simulink model "TLC_Network"  (R2022b)
settings: Solver=VariableStepAuto  StartTime=0.0  StopTime=2  RelTol=1e-3
(part 2 of 2)

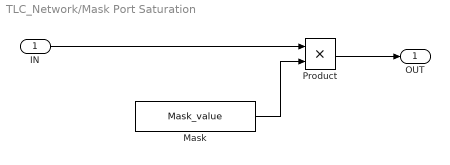
== system TLC_Network/Mask Port Saturation ==
  IN : Inport
  Mask : Constant  Value=Mask_value
  Product : Product
  OUT : Outport
  wires:
  Product/1 -> OUT/1
  IN/1 -> Product/1
  Mask/1 -> Product/2

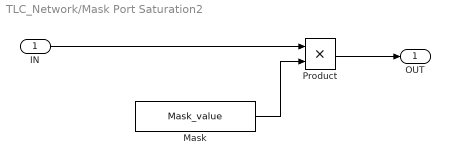
== system TLC_Network/Mask Port Saturation2 ==
  IN : Inport
  Mask : Constant  Value=Mask_value
  Product : Product
  OUT : Outport
  wires:
  Product/1 -> OUT/1
  IN/1 -> Product/1
  Mask/1 -> Product/2

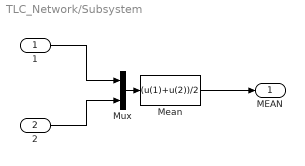
== system TLC_Network/Subsystem ==
  1 : Inport
  2 : Inport  Port=2
  Mean : Fcn  Expr=(u(1)+u(2))/2
  Mux : Mux  Inputs=2
  MEAN : Outport  VectorParamsAs1DForOutWhenUnconnected=off
  wires:
  1/1 -> Mux/1
  Mux/1 -> Mean/1
  2/1 -> Mux/2
  Mean/1 -> MEAN/1

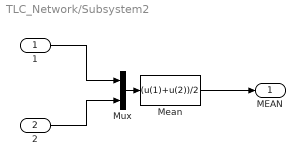
== system TLC_Network/Subsystem2 ==
  1 : Inport
  2 : Inport  Port=2
  Mean : Fcn  Expr=(u(1)+u(2))/2
  Mux : Mux  Inputs=2
  MEAN : Outport  VectorParamsAs1DForOutWhenUnconnected=off
  wires:
  1/1 -> Mux/1
  Mux/1 -> Mean/1
  2/1 -> Mux/2
  Mean/1 -> MEAN/1

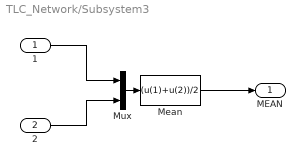
== system TLC_Network/Subsystem3 ==
  1 : Inport
  2 : Inport  Port=2
  Mean : Fcn  Expr=(u(1)+u(2))/2
  Mux : Mux  Inputs=2
  MEAN : Outport  VectorParamsAs1DForOutWhenUnconnected=off
  wires:
  1/1 -> Mux/1
  Mux/1 -> Mean/1
  2/1 -> Mux/2
  Mean/1 -> MEAN/1

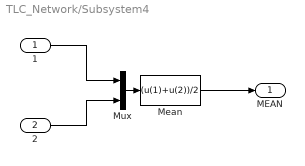
== system TLC_Network/Subsystem4 ==
  1 : Inport
  2 : Inport  Port=2
  Mean : Fcn  Expr=(u(1)+u(2))/2
  Mux : Mux  Inputs=2
  MEAN : Outport  VectorParamsAs1DForOutWhenUnconnected=off
  wires:
  1/1 -> Mux/1
  Mux/1 -> Mean/1
  2/1 -> Mux/2
  Mean/1 -> MEAN/1

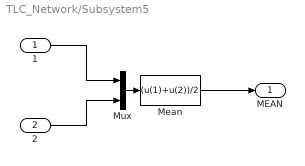
== system TLC_Network/Subsystem5 ==
  1 : Inport
  2 : Inport  Port=2
  Mean : Fcn  Expr=(u(1)+u(2))/2
  Mux : Mux  Inputs=2
  MEAN : Outport  VectorParamsAs1DForOutWhenUnconnected=off
  wires:
  1/1 -> Mux/1
  Mux/1 -> Mean/1
  2/1 -> Mux/2
  Mean/1 -> MEAN/1

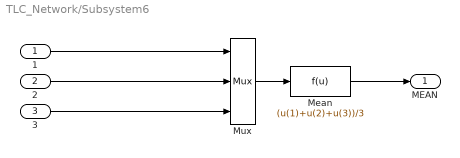
== system TLC_Network/Subsystem6 ==
  1 : Inport
  2 : Inport  Port=2
  3 : Inport  Port=3
  Mean : Fcn  Expr=(u(1)+u(2)+u(3))/3
  Mux : Mux  Inputs=3
  MEAN : Outport  VectorParamsAs1DForOutWhenUnconnected=off
  wires:
  1/1 -> Mux/1
  Mux/1 -> Mean/1
  2/1 -> Mux/2
  Mean/1 -> MEAN/1
  3/1 -> Mux/3

== matlab function TLC_Network/media4 ==
  data: u input; y output
function y = media(u)

y = mean(u);

== matlab function TLC_Network/media5 ==
  data: u input; y output
function y = media(u)

y = mean(u);

== matlab function TLC_Network/media6 ==
  data: u input; y output
function y = media(u)

y = mean(u);

== matlab function TLC_Network/media7 ==
  data: u input; y output
function y = media(u)

y = mean(u);

== matlab function TLC_Network/media8 ==
  data: u input; y output
function y = media(u)

y = mean(u);

== matlab function TLC_Network/media3 ==
  data: u input; y output
function y = media(u)

y = mean(u);
